simulink model "carsim_template_v2"  (R2022b)
settings: Solver=ode3  StartTime=0.0  StopTime=10.0  FixedStep=0.001  RelTol=1e-3
settings Model: Creator=ranwe  LastModifiedBy=ranwe

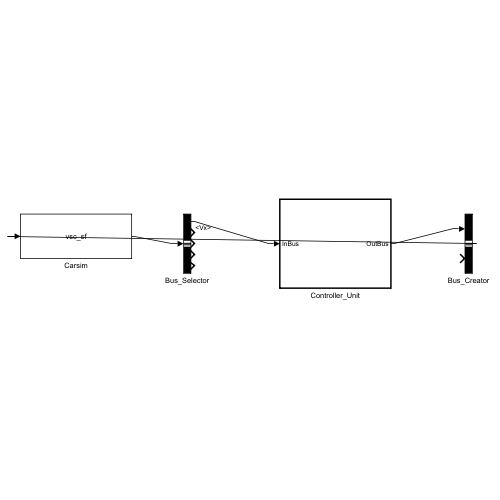
[thumbnail: Simulink's stored preview of the top-level diagram]
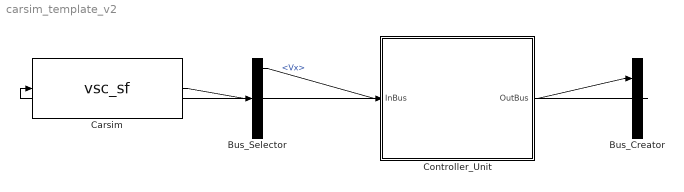
== system carsim_template_v2 ==
  Bus_Creator : BusCreator  Inputs=2  OutDataTypeStr=Bus: Bus_CarSim_In  NonVirtualBus=on
  Bus_Selector : BusSelector  OutputSignals=Vx,Vy,Yaw_Rate,X_O,Y_O
  Carsim : S-Function  FunctionName=vsc_sf  Parameters=simfile.sim  SFunctionDeploymentMode=off  EnableBusSupport=off
  Controller_Unit : Subsystem  TreatAsAtomicUnit=on
  wires:
  Carsim/1 -> Bus_Selector/1
  Bus_Selector/1 -> Controller_Unit/1(InBus)  "<Vx>"
  Controller_Unit/1(OutBus) -> Bus_Creator/1
  Bus_Creator/1 -> Carsim/1

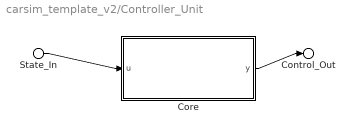
== system carsim_template_v2/Controller_Unit ==
  State_In : Inport  PortName=InBus  Element=Vx
  Core : MATLAB Function  TreatAsAtomicUnit=on
  Control_Out : Outport  PortName=OutBus  Element=Steer_SW
  wires:
  State_In/1 -> Core/1(u)
  Core/1(y) -> Control_Out/1

== matlab function carsim_template_v2/Controller_Unit/Core ==
  data: u input; y output
function y = fcn(u)

y = u;
